simulink model "reg2pol"  (R2021b)
settings: Solver=VariableStepAuto  StartTime=0.0  StopTime=20  RelTol=1e-3
values from neighbouring files (symbols this model uses):
  h = 0.1    [draw_nyquist_and_step.m]    (also in sim_outs.mat = 0.05)
undefined symbols (not defined in the file or in its folder): ym
settings Model: Creator=roman  LastModifiedBy=roman

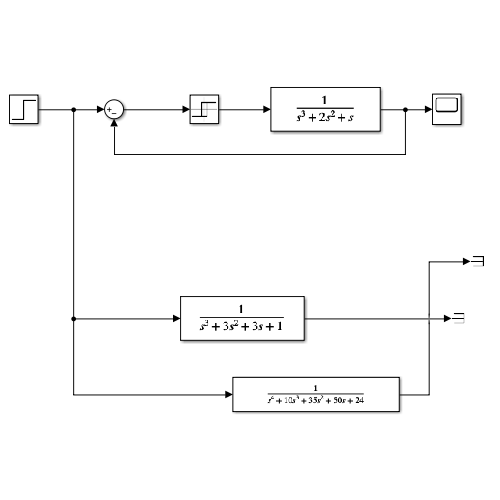
[thumbnail: Simulink's stored preview of the top-level diagram]
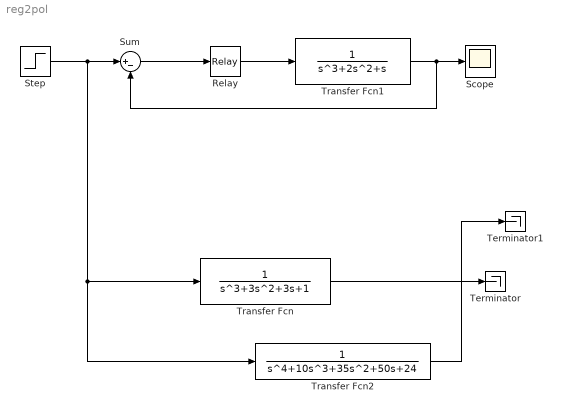
== system reg2pol ==
  Relay : Relay  OnSwitchValue=h  OffSwitchValue=-h  OnOutputValue=ym  OffOutputValue=-ym  ZeroCross=off
  Scope : Scope
  Step : Step  SampleTime=0
  Sum : Sum  Inputs=|+-
  Terminator : Terminator
  Terminator1 : Terminator
  Transfer Fcn : TransferFcn  Denominator=[1 3 3 1]
  Transfer Fcn1 : TransferFcn  Denominator=[1 2 1 0]
  Transfer Fcn2 : TransferFcn  Denominator=[1 10 35 50 24]
  wires:
  Sum/1 -> Relay/1
  Transfer Fcn/1 -> Terminator/1
  Step/1 -> Transfer Fcn2/1, Transfer Fcn/1, Sum/1
  Transfer Fcn2/1 -> Terminator1/1
  Transfer Fcn1/1 -> Sum/2, Scope/1
  Relay/1 -> Transfer Fcn1/1
